simulink model "SERVICEECUsimlik"  (R2024a)
settings: Solver=VariableStepAuto  StartTime=0.0  StopTime=inf  RelTol=1e-3
settings Model: ExtModeTrigDuration=100  Creator=ABDERRAZEK  LastModifiedBy=ABDERRAZEK
settings DataIOCC: StateSaveName=tmp_raccel_xout
settings OptimizationCC: ZeroExternalMemoryAtStartup=off  ZeroInternalMemoryAtStartup=off  EfficientMapNaN2IntZero=off
settings SFSimCC: SimCustomCompilerFlags=-std=c++17  SimTargetLang=C++
settings RTWCC: CustomBLASCallback=coder.internal.blas.MATLABBLASCallback  TargetLang=C++  DLTargetLibrary=mkl-dnn
settings CodeAppCC: GenerateComments=off  MangleLength=10  SimulinkBlockComments=off
settings GRTTargetCC: TargetLangStandard=C++11 (ISO)  CodeInterfacePackaging=C++ class

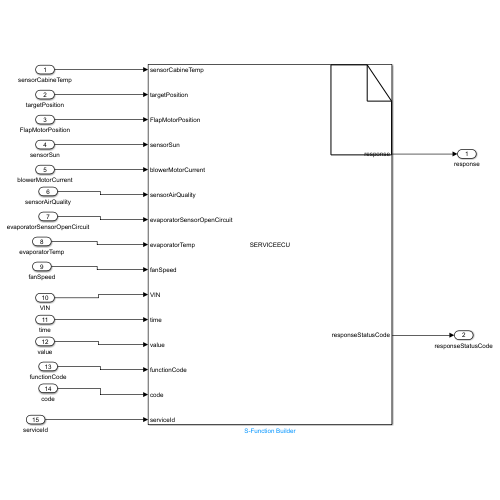
[thumbnail: Simulink's stored preview of the top-level diagram]
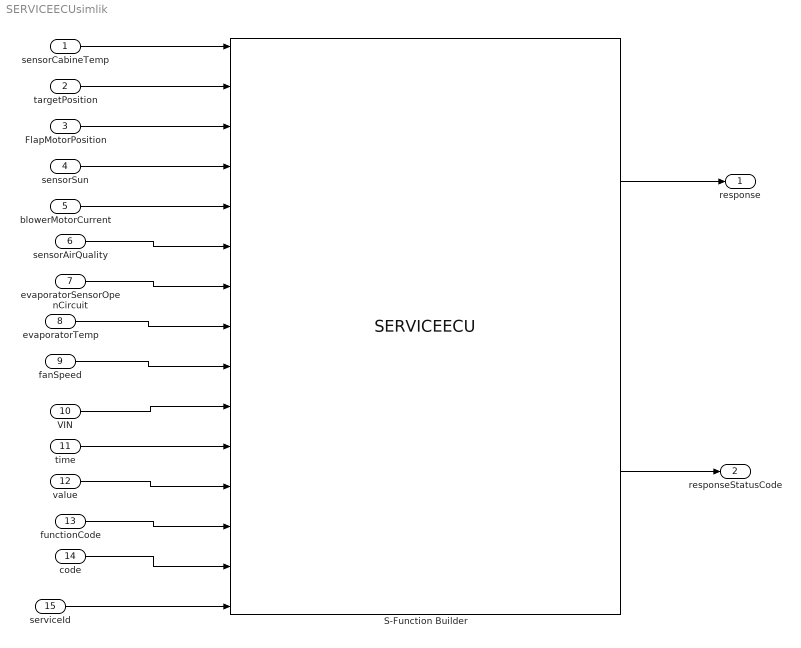
== system SERVICEECUsimlik ==
  sensorCabineTemp : Inport
  targetPosition : Inport  Port=2
  FlapMotorPosition : Inport  Port=3
  sensorSun : Inport  Port=4
  blowerMotorCurrent : Inport  Port=5
  sensorAirQuality : Inport  Port=6
  evaporatorSensorOpenCircuit : Inport  Port=7
  evaporatorTemp : Inport  Port=8
  fanSpeed : Inport  Port=9
  VIN : Inport  Port=10
  time : Inport  Port=11
  value : Inport  Port=12
  functionCode : Inport  Port=13
  code : Inport  Port=14
  serviceId : Inport  Port=15
  S-Function Builder : S-Function  FunctionName=SERVICEECU  SFunctionModules=SERVICEECU_wrapper.cpp  SFunctionDeploymentMode=off  EnableBusSupport=off  mask(S-Function Builder){}
      mask help: Simulink:masks:SFunctionBuilder_MD
      mask init:
      | val = [[.9  0.75 0.75 1 1 .9 .9 1]',[1 1 0.75 0.75 .9 .9 1 .9]'];try , sys = get_param(gcb,'SfunBuilderFcnName');if isempty(sys), sys = get_param(gcb,'FunctionName'); end,catch, sys = get_param(gcb,'FunctionName'); end
      settings: CopyFcn=set_param(gcbh,'LinkStatus','none')  OpenFcn=sfunctionwizard(gcbh)
      mask Display: plot(val(:,1),val(:,2)),disp(sys),port_label('input',1,'sensorCabineTemp'),port_label('input',2,'targetPosition'),port_label('input',3,'FlapMotorPosition'),port_label('input',4,'sensorSun'),port_label('input',5,'blowerMotorCurrent'),port_label('input',6,'sensorAirQuality'),port_label('input',7,'evaporatorSensorOpenCircuit'),port_label('input',8,'evaporatorTemp'),port_label('input',9,'fanSpeed'),port_label('input',10,'VIN'),port_label('input',11,'time'),port_label('input',12,'value'),port_label('input',13,'functionCode'),port_label('input',14,'code'),port_label('input',15,'serviceId'),port_label('output',1,'response'),port_label('output',2,'responseStatusCode')
  response : Outport
  responseStatusCode : Outport  Port=2
  wires:
  sensorCabineTemp/1 -> S-Function Builder/1
  code/1 -> S-Function Builder/14
  functionCode/1 -> S-Function Builder/13
  value/1 -> S-Function Builder/12
  time/1 -> S-Function Builder/11
  VIN/1 -> S-Function Builder/10
  fanSpeed/1 -> S-Function Builder/9
  evaporatorTemp/1 -> S-Function Builder/8
  evaporatorSensorOpenCircuit/1 -> S-Function Builder/7
  sensorAirQuality/1 -> S-Function Builder/6
  blowerMotorCurrent/1 -> S-Function Builder/5
  sensorSun/1 -> S-Function Builder/4
  FlapMotorPosition/1 -> S-Function Builder/3
  targetPosition/1 -> S-Function Builder/2
  S-Function Builder/1 -> response/1
  S-Function Builder/2 -> responseStatusCode/1
  serviceId/1 -> S-Function Builder/15
